simulink model "simsol"  (R2019b)
settings: Solver=VariableStepAuto  StartTime=0.0  StopTime=2  RelTol=1e-3
settings Model: Creator=axs2437  LastModifiedBy=axs2437
settings SolverCC: ZeroCrossAlgorithm=Adaptive
settings DebuggingCC: IgnoredZcDiagnostic=none

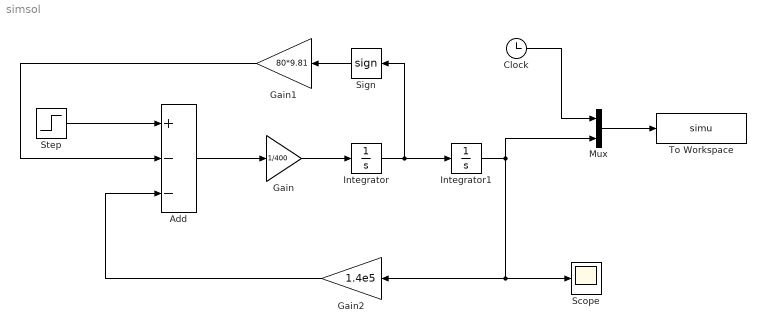
== system simsol ==
  Add : Sum  Inputs=+--
  Clock : Clock
  Gain : Gain  Gain=1/400
  Gain1 : Gain  Gain=80*9.81
  Gain2 : Gain  Gain=1.4e5
  Integrator : Integrator
  Integrator1 : Integrator
  Mux : Mux  Inputs=2
  Scope : Scope
  Sign : Signum
  Step : Step  Time=0  After=1.4e4  SampleTime=0.01
  To Workspace : ToWorkspace  VariableName=simu  SampleTime=-1
  wires:
  Step/1 -> Add/1
  Gain2/1 -> Add/3
  Add/1 -> Gain/1
  Gain/1 -> Integrator/1
  Integrator/1 -> Sign/1, Integrator1/1
  Gain1/1 -> Add/2
  Sign/1 -> Gain1/1
  Integrator1/1 -> Scope/1, Gain2/1, Mux/2
  Clock/1 -> Mux/1
  Mux/1 -> To Workspace/1
